simulink model "simulation"  (R2013a)
settings: Solver=ode45  StartTime=0.0  StopTime=10.0  RelTol=1e-3
libraries: elec_lib x72, nesl_utility x5, fl_lib x4, simulink x3, powerlib x1
settings Model: Creator=Fuad  LastModifiedBy=Fuad

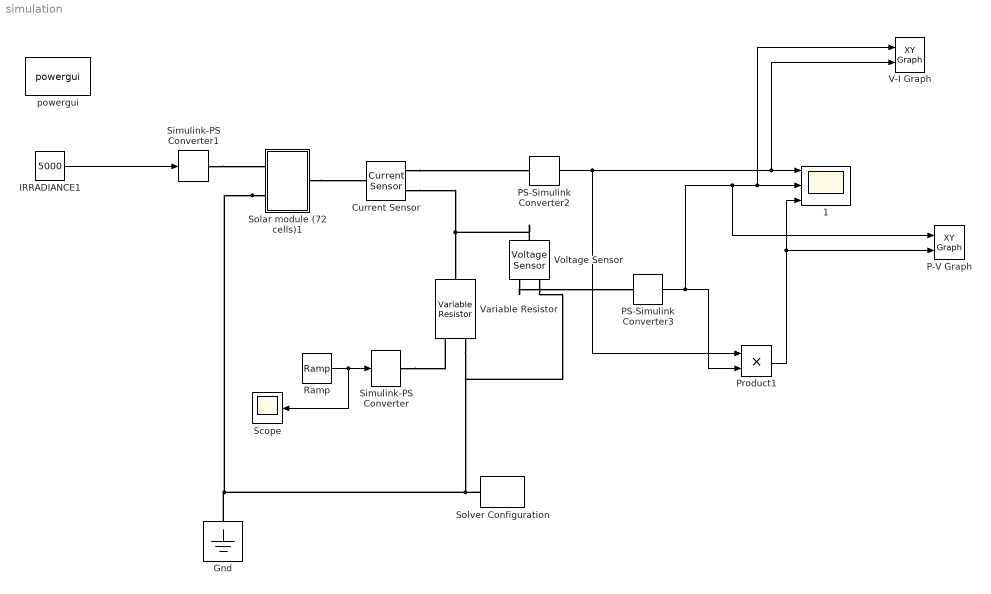
== system simulation ==
  " 1" : Scope  NumInputPorts=3
      settings: TickLabels=on  TimeRange=10  YMin=-5~-5~-5  YMax=5~5~5  SaveName=Sc
  Current Sensor : fl_lib/Electrical/Electrical Sensors/Current Sensor  i1_Log=off  v1_Log=off  LocalVarNames=|i1|v1  LocalVarDescs=|i1|v1  LocalVarLogging=[0 0]
  Gnd : fl_lib/Electrical/Electrical Elements/Electrical Reference  i_Log=off  LocalVarNames=|i  LocalVarDescs=|i  LocalVarLogging=0
  IRRADIANCE1 : Constant  Value=5000
  "P-V Graph " : simulink/Sinks/XY Graph  xmin=0  xmax=50  ymin=0  ymax=900  st=1
  PS-Simulink Converter2 : nesl_utility/PS-Simulink Converter  PhysicalDomain=network_engine_domain  SubClassName=ps_output  LeftPortType=input  RightPortType=output  PseudoPeriodic=off  Frequencies=[]  Unit=1  AffineConversion=off
  PS-Simulink Converter3 : nesl_utility/PS-Simulink Converter  PhysicalDomain=network_engine_domain  SubClassName=ps_output  LeftPortType=input  RightPortType=output  PseudoPeriodic=off  Frequencies=[]  Unit=1  AffineConversion=off
  Product1 : Product
  Ramp : simulink/Sources/Ramp  slope=1  start=0  X0=0
  Scope : Scope
  Simulink-PS Converter : nesl_utility/Simulink-PS Converter  PhysicalDomain=network_engine_domain  SubClassName=ps_input  LeftPortType=input  RightPortType=output  PseudoPeriodic=off  Frequencies=[]  NoiseDistribution=none  NoiseParameters=[]  Unit=1  AffineConversion=off  InputFiltering=on  SimscapeFilterOrder=1  InputFilterTimeConstant=0.001  UdotUserProvided=1
  Simulink-PS Converter1 : nesl_utility/Simulink-PS Converter  PhysicalDomain=network_engine_domain  SubClassName=ps_input  LeftPortType=input  RightPortType=output  PseudoPeriodic=off  Frequencies=[]  NoiseDistribution=none  NoiseParameters=[]  Unit=1  AffineConversion=off  InputFiltering=off  SimscapeFilterOrder=1  InputFilterTimeConstant=.001  UdotUserProvided=0
  Solar module (72 cells)1 : Subsystem
  Solver Configuration : nesl_utility/Solver Configuration  PhysicalDomain=network_engine_domain  SubClassName=solver  LeftPortType=input  RightPortType=generic  Accelerate=off  Tones=[]  Harmonics=[]  SimulateNoise=off  Profile=off  UseLocalSampling=off  EnableSwitchedLinearOptims=on  FrequencyDomain=off  UseCCode=off  UseNewInitialization=off  DoDC=off  ResidualTolerance=1e-09  UseLocalSolver=off  LocalSolverChoice=NE_BACKWARD_EULER_ADVANCER  LocalSolverSampleTime=0.001  DoFixedCost=off  MaxNonlinIter=3  MaxModeIter=2  LinearAlgebra=Sparse  DelaysMemoryBudget=1024
  "V-I Graph " : simulink/Sinks/XY Graph  xmin=0  xmax=50  ymin=0  ymax=100  st=1
  Variable Resistor : fl_lib/Electrical/Electrical Elements/Variable Resistor  Rmin=0 Ohm  i_Log=off  v_Log=off  LocalVarNames=|i|v  LocalVarDescs=|i|v  LocalVarLogging=[0 0]
  Voltage Sensor : fl_lib/Electrical/Electrical Sensors/Voltage Sensor  i1_Log=off  v1_Log=off  LocalVarNames=|i1|v1  LocalVarDescs=|i1|v1  LocalVarLogging=[0 0]
  powergui : powerlib/powergui  Priority=1  SimulationMode=Continuous  SolverType=Tustin  SampleTime=50e-6  frequency=60  SPID=off  DisableSnubberDevices=off  DisableRonSwitches=off  DisableVfSwitches=off  SwTol=0  Interpol=off  DisplayEquations=off  frequencyindice=0  Pbase=100e6  ErrMax=1e-4  Iterations=50  UnitsV=kV  UnitsW=MW  FunctionMessages=off  echomessages=off  HookPort=off  EnableUseOfTLC=off  x0status=blocks  RestoreLinks=warning  ResistiveCurrentMeasurement=off  Frange=[0:2:500]  Ylog=off  Xlog=on  ShowGrid=off  save=off  variable=ZData  ZoomFFT=off  StartTime=0.0  cycles=1  DisplayStyle=1  fundamental=60  FreqAxis=off  MaxFrequency=1000  frequencyindicesteady=1  RmsSteady=1  display=off  Ts=0  methode=off
  wires:
  IRRADIANCE1/1 -> Simulink-PS Converter1/1
  PS-Simulink Converter2/1 -> Product1/1, "V-I Graph "/2, " 1"/1
  Ramp/1 -> Scope/1, Simulink-PS Converter/1
  Product1/1 -> "P-V Graph "/2, " 1"/3
  PS-Simulink Converter3/1 -> "P-V Graph "/1, "V-I Graph "/1, " 1"/2, Product1/2
  connections:
  Solar module (72 cells)1/LConn2 -- Voltage Sensor/RConn2 -- Variable Resistor/LConn2 -- Solver Configuration/RConn1 -- Gnd/LConn1
  Current Sensor/RConn2 -- Voltage Sensor/LConn1 -- Variable Resistor/RConn1
  Simulink-PS Converter1/RConn1 -- Solar module (72 cells)1/LConn1
  Solar module (72 cells)1/RConn1 -- Current Sensor/LConn1
  Simulink-PS Converter/RConn1 -- Variable Resistor/LConn1
  Current Sensor/RConn1 -- PS-Simulink Converter2/LConn1
  Voltage Sensor/RConn1 -- PS-Simulink Converter3/LConn1

== system simulation/Solar module (72 cells)1 ==
  36 solarceel : Subsystem
  36 solarceel1 : Subsystem
  Ir : PMIOPort  Port=1  Side=Left
  + : PMIOPort  Port=2  Side=Right
  - : PMIOPort  Port=3  Side=Left
  connections:
  Ir/RConn1 -- 36 solarceel/LConn1 -- 36 solarceel1/LConn1
  36 solarceel/RConn1 -- 36 solarceel1/LConn2
  +/RConn1 -- 36 solarceel1/RConn1
  -/RConn1 -- 36 solarceel/LConn2

== system simulation/Solar module (72 cells)1/36 solarceel ==
  18 solar cells : Subsystem
  18 solar cells1 : Subsystem
  Ir : PMIOPort  Port=1  Side=Left
  + : PMIOPort  Port=2  Side=Right
  - : PMIOPort  Port=3  Side=Left
  connections:
  Ir/RConn1 -- 18 solar cells1/LConn1 -- 18 solar cells/LConn1
  18 solar cells/RConn1 -- 18 solar cells1/LConn2
  +/RConn1 -- 18 solar cells1/RConn1
  -/RConn1 -- 18 solar cells/LConn2

== system simulation/Solar module (72 cells)1/36 solarceel1 ==
  18 solar cells : Subsystem
  18 solar cells1 : Subsystem
  Ir : PMIOPort  Port=1  Side=Left
  + : PMIOPort  Port=2  Side=Right
  - : PMIOPort  Port=3  Side=Left
  connections:
  18 solar cells/LConn1 -- Ir/RConn1 -- 18 solar cells1/LConn1
  18 solar cells/RConn1 -- 18 solar cells1/LConn2
  +/RConn1 -- 18 solar cells1/RConn1
  -/RConn1 -- 18 solar cells/LConn2

== system simulation/Solar module (72 cells)1/36 solarceel/18 solar cells ==
  6solarcells : Subsystem
  6solarcells1 : Subsystem
  6solarcells2 : Subsystem
  + : PMIOPort  Port=1  Side=Right
  Ir : PMIOPort  Port=2  Side=Left
  - : PMIOPort  Port=3  Side=Left
  connections:
  Ir/RConn1 -- 6solarcells1/LConn1 -- 6solarcells/LConn1 -- 6solarcells2/LConn1
  6solarcells/RConn1 -- 6solarcells1/LConn2
  6solarcells1/RConn1 -- 6solarcells2/LConn2
  +/RConn1 -- 6solarcells2/RConn1
  -/RConn1 -- 6solarcells/LConn2

== system simulation/Solar module (72 cells)1/36 solarceel/18 solar cells1 ==
  6solarcells : Subsystem
  6solarcells1 : Subsystem
  6solarcells2 : Subsystem
  + : PMIOPort  Port=1  Side=Right
  Ir : PMIOPort  Port=2  Side=Left
  - : PMIOPort  Port=3  Side=Left
  connections:
  6solarcells1/LConn1 -- 6solarcells/LConn1 -- Ir/RConn1 -- 6solarcells2/LConn1
  6solarcells/RConn1 -- 6solarcells1/LConn2
  6solarcells1/RConn1 -- 6solarcells2/LConn2
  +/RConn1 -- 6solarcells2/RConn1
  -/RConn1 -- 6solarcells/LConn2

== system simulation/Solar module (72 cells)1/36 solarceel1/18 solar cells ==
  6solarcells : Subsystem
  6solarcells1 : Subsystem
  6solarcells2 : Subsystem
  + : PMIOPort  Port=1  Side=Right
  Ir : PMIOPort  Port=2  Side=Left
  - : PMIOPort  Port=3  Side=Left
  connections:
  6solarcells1/LConn1 -- 6solarcells/LConn1 -- Ir/RConn1 -- 6solarcells2/LConn1
  6solarcells/RConn1 -- 6solarcells1/LConn2
  6solarcells1/RConn1 -- 6solarcells2/LConn2
  +/RConn1 -- 6solarcells2/RConn1
  -/RConn1 -- 6solarcells/LConn2

== system simulation/Solar module (72 cells)1/36 solarceel1/18 solar cells1 ==
  6solarcells : Subsystem
  6solarcells1 : Subsystem
  6solarcells2 : Subsystem
  + : PMIOPort  Port=1  Side=Right
  Ir : PMIOPort  Port=2  Side=Left
  - : PMIOPort  Port=3  Side=Left
  connections:
  6solarcells1/LConn1 -- 6solarcells/LConn1 -- Ir/RConn1 -- 6solarcells2/LConn1
  6solarcells/RConn1 -- 6solarcells1/LConn2
  6solarcells1/RConn1 -- 6solarcells2/LConn2
  +/RConn1 -- 6solarcells2/RConn1
  -/RConn1 -- 6solarcells/LConn2

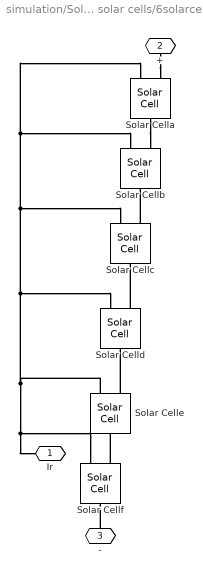
== system simulation/Solar module (72 cells)1/36 solarceel/18 solar cells/6solarcells ==
  Solar Cella : elec_lib/Sources/Solar Cell  prm=1  Isc=4.75 A  Voc=0.6 V  Is=1e-6 A  Is2=0 A  Iph=7.34 A  Ir0=1000 W/m^2  ec=1.6  N2=2  Rs=5.1e-3 Ohm  Rp=Inf Ohm  TIPH1=0.65e-3 1/K  EG=1.12 eV  TXIS1=3  TXIS2=3  TRS1=0  TRP1=0  Tmeas=25 C  TFIXED=25 C  LocalVarLogging=[]  thermal_mass=100 J/K  initial_temperature=25 C
  Solar Cellb : elec_lib/Sources/Solar Cell  prm=1  Isc=4.75 A  Voc=0.6 V  Is=1e-6 A  Is2=0 A  Iph=7.34 A  Ir0=1000 W/m^2  ec=1.6  N2=2  Rs=5.1e-3 Ohm  Rp=Inf Ohm  TIPH1=0.65e-3 1/K  EG=1.12 eV  TXIS1=3  TXIS2=3  TRS1=0  TRP1=0  Tmeas=25 C  TFIXED=25 C  LocalVarLogging=[]  thermal_mass=100 J/K  initial_temperature=25 C
  Solar Cellc : elec_lib/Sources/Solar Cell  prm=1  Isc=4.75 A  Voc=0.6 V  Is=1e-6 A  Is2=0 A  Iph=7.34 A  Ir0=1000 W/m^2  ec=1.6  N2=2  Rs=5.1e-3 Ohm  Rp=Inf Ohm  TIPH1=0.65e-3 1/K  EG=1.12 eV  TXIS1=3  TXIS2=3  TRS1=0  TRP1=0  Tmeas=25 C  TFIXED=25 C  LocalVarLogging=[]  thermal_mass=100 J/K  initial_temperature=25 C
  Solar Celld : elec_lib/Sources/Solar Cell  prm=1  Isc=4.75 A  Voc=0.6 V  Is=1e-6 A  Is2=0 A  Iph=7.34 A  Ir0=1000 W/m^2  ec=1.6  N2=2  Rs=5.1e-3 Ohm  Rp=Inf Ohm  TIPH1=0.65e-3 1/K  EG=1.12 eV  TXIS1=3  TXIS2=3  TRS1=0  TRP1=0  Tmeas=25 C  TFIXED=25 C  LocalVarLogging=[]  thermal_mass=100 J/K  initial_temperature=25 C
  Solar Celle : elec_lib/Sources/Solar Cell  prm=1  Isc=4.75 A  Voc=0.6 V  Is=1e-6 A  Is2=0 A  Iph=7.34 A  Ir0=1000 W/m^2  ec=1.6  N2=2  Rs=5.1e-3 Ohm  Rp=Inf Ohm  TIPH1=0.65e-3 1/K  EG=1.12 eV  TXIS1=3  TXIS2=3  TRS1=0  TRP1=0  Tmeas=25 C  TFIXED=25 C  LocalVarLogging=[]  thermal_mass=100 J/K  initial_temperature=25 C
  Solar Cellf : elec_lib/Sources/Solar Cell  prm=1  Isc=4.75 A  Voc=0.6 V  Is=1e-6 A  Is2=0 A  Iph=7.34 A  Ir0=1000 W/m^2  ec=1.6  N2=2  Rs=5.1e-3 Ohm  Rp=Inf Ohm  TIPH1=0.65e-3 1/K  EG=1.12 eV  TXIS1=3  TXIS2=3  TRS1=0  TRP1=0  Tmeas=25 C  TFIXED=25 C  LocalVarLogging=[]  thermal_mass=100 J/K  initial_temperature=25 C
  Ir : PMIOPort  Port=1  Side=Left
  + : PMIOPort  Port=2  Side=Right
  - : PMIOPort  Port=3  Side=Left
  connections:
  Ir/RConn1 -- Solar Celle/LConn1 -- Solar Celld/LConn1 -- Solar Cellc/LConn1 -- Solar Cellb/LConn1 -- Solar Cella/LConn1 -- Solar Cellf/LConn1
  Solar Cella/RConn1 -- Solar Cellb/LConn2
  Solar Cellc/LConn2 -- Solar Cellb/RConn1
  Solar Celld/LConn2 -- Solar Cellc/RConn1
  Solar Celle/LConn2 -- Solar Celld/RConn1
  Solar Cellf/LConn2 -- Solar Celle/RConn1
  +/RConn1 -- Solar Cella/LConn2
  -/RConn1 -- Solar Cellf/RConn1

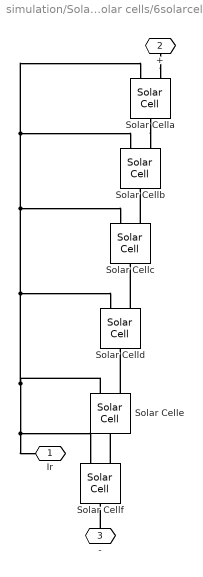
== system simulation/Solar module (72 cells)1/36 solarceel/18 solar cells/6solarcells1 ==
  Solar Cella : elec_lib/Sources/Solar Cell  prm=1  Isc=4.75 A  Voc=0.6 V  Is=1e-6 A  Is2=0 A  Iph=7.34 A  Ir0=1000 W/m^2  ec=1.6  N2=2  Rs=5.1e-3 Ohm  Rp=Inf Ohm  TIPH1=0.65e-3 1/K  EG=1.12 eV  TXIS1=3  TXIS2=3  TRS1=0  TRP1=0  Tmeas=25 C  TFIXED=25 C  LocalVarLogging=[]  thermal_mass=100 J/K  initial_temperature=25 C
  Solar Cellb : elec_lib/Sources/Solar Cell  prm=1  Isc=4.75 A  Voc=0.6 V  Is=1e-6 A  Is2=0 A  Iph=7.34 A  Ir0=1000 W/m^2  ec=1.6  N2=2  Rs=5.1e-3 Ohm  Rp=Inf Ohm  TIPH1=0.65e-3 1/K  EG=1.12 eV  TXIS1=3  TXIS2=3  TRS1=0  TRP1=0  Tmeas=25 C  TFIXED=25 C  LocalVarLogging=[]  thermal_mass=100 J/K  initial_temperature=25 C
  Solar Cellc : elec_lib/Sources/Solar Cell  prm=1  Isc=4.75 A  Voc=0.6 V  Is=1e-6 A  Is2=0 A  Iph=7.34 A  Ir0=1000 W/m^2  ec=1.6  N2=2  Rs=5.1e-3 Ohm  Rp=Inf Ohm  TIPH1=0.65e-3 1/K  EG=1.12 eV  TXIS1=3  TXIS2=3  TRS1=0  TRP1=0  Tmeas=25 C  TFIXED=25 C  LocalVarLogging=[]  thermal_mass=100 J/K  initial_temperature=25 C
  Solar Celld : elec_lib/Sources/Solar Cell  prm=1  Isc=4.75 A  Voc=0.6 V  Is=1e-6 A  Is2=0 A  Iph=7.34 A  Ir0=1000 W/m^2  ec=1.6  N2=2  Rs=5.1e-3 Ohm  Rp=Inf Ohm  TIPH1=0.65e-3 1/K  EG=1.12 eV  TXIS1=3  TXIS2=3  TRS1=0  TRP1=0  Tmeas=25 C  TFIXED=25 C  LocalVarLogging=[]  thermal_mass=100 J/K  initial_temperature=25 C
  Solar Celle : elec_lib/Sources/Solar Cell  prm=1  Isc=4.75 A  Voc=0.6 V  Is=1e-6 A  Is2=0 A  Iph=7.34 A  Ir0=1000 W/m^2  ec=1.6  N2=2  Rs=5.1e-3 Ohm  Rp=Inf Ohm  TIPH1=0.65e-3 1/K  EG=1.12 eV  TXIS1=3  TXIS2=3  TRS1=0  TRP1=0  Tmeas=25 C  TFIXED=25 C  LocalVarLogging=[]  thermal_mass=100 J/K  initial_temperature=25 C
  Solar Cellf : elec_lib/Sources/Solar Cell  prm=1  Isc=4.75 A  Voc=0.6 V  Is=1e-6 A  Is2=0 A  Iph=7.34 A  Ir0=1000 W/m^2  ec=1.6  N2=2  Rs=5.1e-3 Ohm  Rp=Inf Ohm  TIPH1=0.65e-3 1/K  EG=1.12 eV  TXIS1=3  TXIS2=3  TRS1=0  TRP1=0  Tmeas=25 C  TFIXED=25 C  LocalVarLogging=[]  thermal_mass=100 J/K  initial_temperature=25 C
  Ir : PMIOPort  Port=1  Side=Left
  + : PMIOPort  Port=2  Side=Right
  - : PMIOPort  Port=3  Side=Left
  connections:
  Solar Celle/LConn1 -- Solar Cellf/LConn1 -- Ir/RConn1 -- Solar Celld/LConn1 -- Solar Cellc/LConn1 -- Solar Cella/LConn1 -- Solar Cellb/LConn1
  Solar Cella/RConn1 -- Solar Cellb/LConn2
  Solar Cellc/LConn2 -- Solar Cellb/RConn1
  Solar Celld/LConn2 -- Solar Cellc/RConn1
  Solar Celle/LConn2 -- Solar Celld/RConn1
  Solar Cellf/LConn2 -- Solar Celle/RConn1
  +/RConn1 -- Solar Cella/LConn2
  -/RConn1 -- Solar Cellf/RConn1

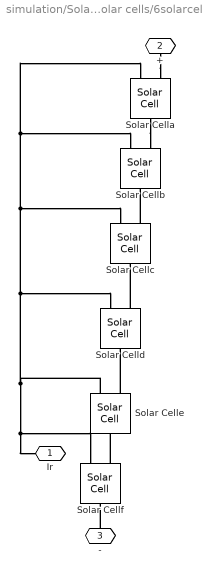
== system simulation/Solar module (72 cells)1/36 solarceel/18 solar cells/6solarcells2 ==
  Solar Cella : elec_lib/Sources/Solar Cell  prm=1  Isc=4.75 A  Voc=0.6 V  Is=1e-6 A  Is2=0 A  Iph=7.34 A  Ir0=1000 W/m^2  ec=1.6  N2=2  Rs=5.1e-3 Ohm  Rp=Inf Ohm  TIPH1=0.65e-3 1/K  EG=1.12 eV  TXIS1=3  TXIS2=3  TRS1=0  TRP1=0  Tmeas=25 C  TFIXED=25 C  LocalVarLogging=[]  thermal_mass=100 J/K  initial_temperature=25 C
  Solar Cellb : elec_lib/Sources/Solar Cell  prm=1  Isc=4.75 A  Voc=0.6 V  Is=1e-6 A  Is2=0 A  Iph=7.34 A  Ir0=1000 W/m^2  ec=1.6  N2=2  Rs=5.1e-3 Ohm  Rp=Inf Ohm  TIPH1=0.65e-3 1/K  EG=1.12 eV  TXIS1=3  TXIS2=3  TRS1=0  TRP1=0  Tmeas=25 C  TFIXED=25 C  LocalVarLogging=[]  thermal_mass=100 J/K  initial_temperature=25 C
  Solar Cellc : elec_lib/Sources/Solar Cell  prm=1  Isc=4.75 A  Voc=0.6 V  Is=1e-6 A  Is2=0 A  Iph=7.34 A  Ir0=1000 W/m^2  ec=1.6  N2=2  Rs=5.1e-3 Ohm  Rp=Inf Ohm  TIPH1=0.65e-3 1/K  EG=1.12 eV  TXIS1=3  TXIS2=3  TRS1=0  TRP1=0  Tmeas=25 C  TFIXED=25 C  LocalVarLogging=[]  thermal_mass=100 J/K  initial_temperature=25 C
  Solar Celld : elec_lib/Sources/Solar Cell  prm=1  Isc=4.75 A  Voc=0.6 V  Is=1e-6 A  Is2=0 A  Iph=7.34 A  Ir0=1000 W/m^2  ec=1.6  N2=2  Rs=5.1e-3 Ohm  Rp=Inf Ohm  TIPH1=0.65e-3 1/K  EG=1.12 eV  TXIS1=3  TXIS2=3  TRS1=0  TRP1=0  Tmeas=25 C  TFIXED=25 C  LocalVarLogging=[]  thermal_mass=100 J/K  initial_temperature=25 C
  Solar Celle : elec_lib/Sources/Solar Cell  prm=1  Isc=4.75 A  Voc=0.6 V  Is=1e-6 A  Is2=0 A  Iph=7.34 A  Ir0=1000 W/m^2  ec=1.6  N2=2  Rs=5.1e-3 Ohm  Rp=Inf Ohm  TIPH1=0.65e-3 1/K  EG=1.12 eV  TXIS1=3  TXIS2=3  TRS1=0  TRP1=0  Tmeas=25 C  TFIXED=25 C  LocalVarLogging=[]  thermal_mass=100 J/K  initial_temperature=25 C
  Solar Cellf : elec_lib/Sources/Solar Cell  prm=1  Isc=4.75 A  Voc=0.6 V  Is=1e-6 A  Is2=0 A  Iph=7.34 A  Ir0=1000 W/m^2  ec=1.6  N2=2  Rs=5.1e-3 Ohm  Rp=Inf Ohm  TIPH1=0.65e-3 1/K  EG=1.12 eV  TXIS1=3  TXIS2=3  TRS1=0  TRP1=0  Tmeas=25 C  TFIXED=25 C  LocalVarLogging=[]  thermal_mass=100 J/K  initial_temperature=25 C
  Ir : PMIOPort  Port=1  Side=Left
  + : PMIOPort  Port=2  Side=Right
  - : PMIOPort  Port=3  Side=Left
  connections:
  Solar Celle/LConn1 -- Solar Cellf/LConn1 -- Ir/RConn1 -- Solar Celld/LConn1 -- Solar Cellc/LConn1 -- Solar Cella/LConn1 -- Solar Cellb/LConn1
  Solar Cella/RConn1 -- Solar Cellb/LConn2
  Solar Cellc/LConn2 -- Solar Cellb/RConn1
  Solar Celld/LConn2 -- Solar Cellc/RConn1
  Solar Celle/LConn2 -- Solar Celld/RConn1
  Solar Cellf/LConn2 -- Solar Celle/RConn1
  +/RConn1 -- Solar Cella/LConn2
  -/RConn1 -- Solar Cellf/RConn1

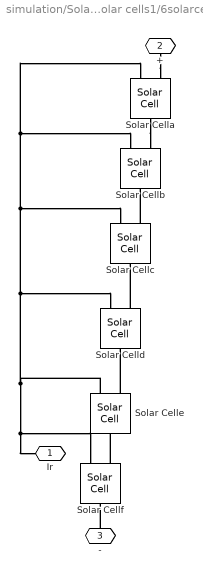
== system simulation/Solar module (72 cells)1/36 solarceel/18 solar cells1/6solarcells ==
  Solar Cella : elec_lib/Sources/Solar Cell  prm=1  Isc=4.75 A  Voc=0.6 V  Is=1e-6 A  Is2=0 A  Iph=7.34 A  Ir0=1000 W/m^2  ec=1.6  N2=2  Rs=5.1e-3 Ohm  Rp=Inf Ohm  TIPH1=0.65e-3 1/K  EG=1.12 eV  TXIS1=3  TXIS2=3  TRS1=0  TRP1=0  Tmeas=25 C  TFIXED=25 C  LocalVarLogging=[]  thermal_mass=100 J/K  initial_temperature=25 C
  Solar Cellb : elec_lib/Sources/Solar Cell  prm=1  Isc=4.75 A  Voc=0.6 V  Is=1e-6 A  Is2=0 A  Iph=7.34 A  Ir0=1000 W/m^2  ec=1.6  N2=2  Rs=5.1e-3 Ohm  Rp=Inf Ohm  TIPH1=0.65e-3 1/K  EG=1.12 eV  TXIS1=3  TXIS2=3  TRS1=0  TRP1=0  Tmeas=25 C  TFIXED=25 C  LocalVarLogging=[]  thermal_mass=100 J/K  initial_temperature=25 C
  Solar Cellc : elec_lib/Sources/Solar Cell  prm=1  Isc=4.75 A  Voc=0.6 V  Is=1e-6 A  Is2=0 A  Iph=7.34 A  Ir0=1000 W/m^2  ec=1.6  N2=2  Rs=5.1e-3 Ohm  Rp=Inf Ohm  TIPH1=0.65e-3 1/K  EG=1.12 eV  TXIS1=3  TXIS2=3  TRS1=0  TRP1=0  Tmeas=25 C  TFIXED=25 C  LocalVarLogging=[]  thermal_mass=100 J/K  initial_temperature=25 C
  Solar Celld : elec_lib/Sources/Solar Cell  prm=1  Isc=4.75 A  Voc=0.6 V  Is=1e-6 A  Is2=0 A  Iph=7.34 A  Ir0=1000 W/m^2  ec=1.6  N2=2  Rs=5.1e-3 Ohm  Rp=Inf Ohm  TIPH1=0.65e-3 1/K  EG=1.12 eV  TXIS1=3  TXIS2=3  TRS1=0  TRP1=0  Tmeas=25 C  TFIXED=25 C  LocalVarLogging=[]  thermal_mass=100 J/K  initial_temperature=25 C
  Solar Celle : elec_lib/Sources/Solar Cell  prm=1  Isc=4.75 A  Voc=0.6 V  Is=1e-6 A  Is2=0 A  Iph=7.34 A  Ir0=1000 W/m^2  ec=1.6  N2=2  Rs=5.1e-3 Ohm  Rp=Inf Ohm  TIPH1=0.65e-3 1/K  EG=1.12 eV  TXIS1=3  TXIS2=3  TRS1=0  TRP1=0  Tmeas=25 C  TFIXED=25 C  LocalVarLogging=[]  thermal_mass=100 J/K  initial_temperature=25 C
  Solar Cellf : elec_lib/Sources/Solar Cell  prm=1  Isc=4.75 A  Voc=0.6 V  Is=1e-6 A  Is2=0 A  Iph=7.34 A  Ir0=1000 W/m^2  ec=1.6  N2=2  Rs=5.1e-3 Ohm  Rp=Inf Ohm  TIPH1=0.65e-3 1/K  EG=1.12 eV  TXIS1=3  TXIS2=3  TRS1=0  TRP1=0  Tmeas=25 C  TFIXED=25 C  LocalVarLogging=[]  thermal_mass=100 J/K  initial_temperature=25 C
  Ir : PMIOPort  Port=1  Side=Left
  + : PMIOPort  Port=2  Side=Right
  - : PMIOPort  Port=3  Side=Left
  connections:
  Solar Celle/LConn1 -- Solar Cellf/LConn1 -- Ir/RConn1 -- Solar Celld/LConn1 -- Solar Cellc/LConn1 -- Solar Cella/LConn1 -- Solar Cellb/LConn1
  Solar Cella/RConn1 -- Solar Cellb/LConn2
  Solar Cellc/LConn2 -- Solar Cellb/RConn1
  Solar Celld/LConn2 -- Solar Cellc/RConn1
  Solar Celle/LConn2 -- Solar Celld/RConn1
  Solar Cellf/LConn2 -- Solar Celle/RConn1
  +/RConn1 -- Solar Cella/LConn2
  -/RConn1 -- Solar Cellf/RConn1

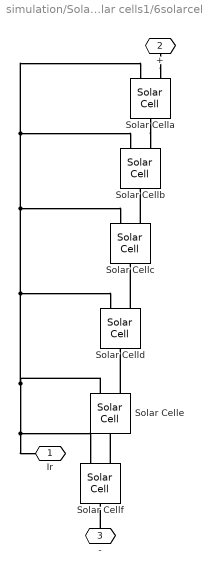
== system simulation/Solar module (72 cells)1/36 solarceel/18 solar cells1/6solarcells1 ==
  Solar Cella : elec_lib/Sources/Solar Cell  prm=1  Isc=4.75 A  Voc=0.6 V  Is=1e-6 A  Is2=0 A  Iph=7.34 A  Ir0=1000 W/m^2  ec=1.6  N2=2  Rs=5.1e-3 Ohm  Rp=Inf Ohm  TIPH1=0.65e-3 1/K  EG=1.12 eV  TXIS1=3  TXIS2=3  TRS1=0  TRP1=0  Tmeas=25 C  TFIXED=25 C  LocalVarLogging=[]  thermal_mass=100 J/K  initial_temperature=25 C
  Solar Cellb : elec_lib/Sources/Solar Cell  prm=1  Isc=4.75 A  Voc=0.6 V  Is=1e-6 A  Is2=0 A  Iph=7.34 A  Ir0=1000 W/m^2  ec=1.6  N2=2  Rs=5.1e-3 Ohm  Rp=Inf Ohm  TIPH1=0.65e-3 1/K  EG=1.12 eV  TXIS1=3  TXIS2=3  TRS1=0  TRP1=0  Tmeas=25 C  TFIXED=25 C  LocalVarLogging=[]  thermal_mass=100 J/K  initial_temperature=25 C
  Solar Cellc : elec_lib/Sources/Solar Cell  prm=1  Isc=4.75 A  Voc=0.6 V  Is=1e-6 A  Is2=0 A  Iph=7.34 A  Ir0=1000 W/m^2  ec=1.6  N2=2  Rs=5.1e-3 Ohm  Rp=Inf Ohm  TIPH1=0.65e-3 1/K  EG=1.12 eV  TXIS1=3  TXIS2=3  TRS1=0  TRP1=0  Tmeas=25 C  TFIXED=25 C  LocalVarLogging=[]  thermal_mass=100 J/K  initial_temperature=25 C
  Solar Celld : elec_lib/Sources/Solar Cell  prm=1  Isc=4.75 A  Voc=0.6 V  Is=1e-6 A  Is2=0 A  Iph=7.34 A  Ir0=1000 W/m^2  ec=1.6  N2=2  Rs=5.1e-3 Ohm  Rp=Inf Ohm  TIPH1=0.65e-3 1/K  EG=1.12 eV  TXIS1=3  TXIS2=3  TRS1=0  TRP1=0  Tmeas=25 C  TFIXED=25 C  LocalVarLogging=[]  thermal_mass=100 J/K  initial_temperature=25 C
  Solar Celle : elec_lib/Sources/Solar Cell  prm=1  Isc=4.75 A  Voc=0.6 V  Is=1e-6 A  Is2=0 A  Iph=7.34 A  Ir0=1000 W/m^2  ec=1.6  N2=2  Rs=5.1e-3 Ohm  Rp=Inf Ohm  TIPH1=0.65e-3 1/K  EG=1.12 eV  TXIS1=3  TXIS2=3  TRS1=0  TRP1=0  Tmeas=25 C  TFIXED=25 C  LocalVarLogging=[]  thermal_mass=100 J/K  initial_temperature=25 C
  Solar Cellf : elec_lib/Sources/Solar Cell  prm=1  Isc=4.75 A  Voc=0.6 V  Is=1e-6 A  Is2=0 A  Iph=7.34 A  Ir0=1000 W/m^2  ec=1.6  N2=2  Rs=5.1e-3 Ohm  Rp=Inf Ohm  TIPH1=0.65e-3 1/K  EG=1.12 eV  TXIS1=3  TXIS2=3  TRS1=0  TRP1=0  Tmeas=25 C  TFIXED=25 C  LocalVarLogging=[]  thermal_mass=100 J/K  initial_temperature=25 C
  Ir : PMIOPort  Port=1  Side=Left
  + : PMIOPort  Port=2  Side=Right
  - : PMIOPort  Port=3  Side=Left
  connections:
  Solar Celle/LConn1 -- Solar Cellf/LConn1 -- Ir/RConn1 -- Solar Celld/LConn1 -- Solar Cellc/LConn1 -- Solar Cella/LConn1 -- Solar Cellb/LConn1
  Solar Cella/RConn1 -- Solar Cellb/LConn2
  Solar Cellc/LConn2 -- Solar Cellb/RConn1
  Solar Celld/LConn2 -- Solar Cellc/RConn1
  Solar Celle/LConn2 -- Solar Celld/RConn1
  Solar Cellf/LConn2 -- Solar Celle/RConn1
  +/RConn1 -- Solar Cella/LConn2
  -/RConn1 -- Solar Cellf/RConn1

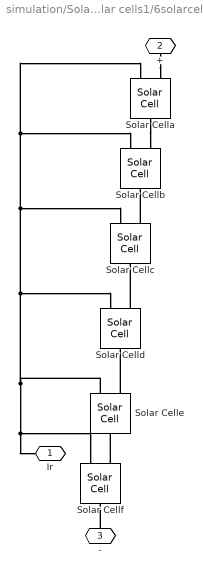
== system simulation/Solar module (72 cells)1/36 solarceel/18 solar cells1/6solarcells2 ==
  Solar Cella : elec_lib/Sources/Solar Cell  prm=1  Isc=4.75 A  Voc=0.6 V  Is=1e-6 A  Is2=0 A  Iph=7.34 A  Ir0=1000 W/m^2  ec=1.6  N2=2  Rs=5.1e-3 Ohm  Rp=Inf Ohm  TIPH1=0.65e-3 1/K  EG=1.12 eV  TXIS1=3  TXIS2=3  TRS1=0  TRP1=0  Tmeas=25 C  TFIXED=25 C  LocalVarLogging=[]  thermal_mass=100 J/K  initial_temperature=25 C
  Solar Cellb : elec_lib/Sources/Solar Cell  prm=1  Isc=4.75 A  Voc=0.6 V  Is=1e-6 A  Is2=0 A  Iph=7.34 A  Ir0=1000 W/m^2  ec=1.6  N2=2  Rs=5.1e-3 Ohm  Rp=Inf Ohm  TIPH1=0.65e-3 1/K  EG=1.12 eV  TXIS1=3  TXIS2=3  TRS1=0  TRP1=0  Tmeas=25 C  TFIXED=25 C  LocalVarLogging=[]  thermal_mass=100 J/K  initial_temperature=25 C
  Solar Cellc : elec_lib/Sources/Solar Cell  prm=1  Isc=4.75 A  Voc=0.6 V  Is=1e-6 A  Is2=0 A  Iph=7.34 A  Ir0=1000 W/m^2  ec=1.6  N2=2  Rs=5.1e-3 Ohm  Rp=Inf Ohm  TIPH1=0.65e-3 1/K  EG=1.12 eV  TXIS1=3  TXIS2=3  TRS1=0  TRP1=0  Tmeas=25 C  TFIXED=25 C  LocalVarLogging=[]  thermal_mass=100 J/K  initial_temperature=25 C
  Solar Celld : elec_lib/Sources/Solar Cell  prm=1  Isc=4.75 A  Voc=0.6 V  Is=1e-6 A  Is2=0 A  Iph=7.34 A  Ir0=1000 W/m^2  ec=1.6  N2=2  Rs=5.1e-3 Ohm  Rp=Inf Ohm  TIPH1=0.65e-3 1/K  EG=1.12 eV  TXIS1=3  TXIS2=3  TRS1=0  TRP1=0  Tmeas=25 C  TFIXED=25 C  LocalVarLogging=[]  thermal_mass=100 J/K  initial_temperature=25 C
  Solar Celle : elec_lib/Sources/Solar Cell  prm=1  Isc=4.75 A  Voc=0.6 V  Is=1e-6 A  Is2=0 A  Iph=7.34 A  Ir0=1000 W/m^2  ec=1.6  N2=2  Rs=5.1e-3 Ohm  Rp=Inf Ohm  TIPH1=0.65e-3 1/K  EG=1.12 eV  TXIS1=3  TXIS2=3  TRS1=0  TRP1=0  Tmeas=25 C  TFIXED=25 C  LocalVarLogging=[]  thermal_mass=100 J/K  initial_temperature=25 C
  Solar Cellf : elec_lib/Sources/Solar Cell  prm=1  Isc=4.75 A  Voc=0.6 V  Is=1e-6 A  Is2=0 A  Iph=7.34 A  Ir0=1000 W/m^2  ec=1.6  N2=2  Rs=5.1e-3 Ohm  Rp=Inf Ohm  TIPH1=0.65e-3 1/K  EG=1.12 eV  TXIS1=3  TXIS2=3  TRS1=0  TRP1=0  Tmeas=25 C  TFIXED=25 C  LocalVarLogging=[]  thermal_mass=100 J/K  initial_temperature=25 C
  Ir : PMIOPort  Port=1  Side=Left
  + : PMIOPort  Port=2  Side=Right
  - : PMIOPort  Port=3  Side=Left
  connections:
  Solar Celle/LConn1 -- Solar Cellf/LConn1 -- Ir/RConn1 -- Solar Celld/LConn1 -- Solar Cellc/LConn1 -- Solar Cella/LConn1 -- Solar Cellb/LConn1
  Solar Cella/RConn1 -- Solar Cellb/LConn2
  Solar Cellc/LConn2 -- Solar Cellb/RConn1
  Solar Celld/LConn2 -- Solar Cellc/RConn1
  Solar Celle/LConn2 -- Solar Celld/RConn1
  Solar Cellf/LConn2 -- Solar Celle/RConn1
  +/RConn1 -- Solar Cella/LConn2
  -/RConn1 -- Solar Cellf/RConn1

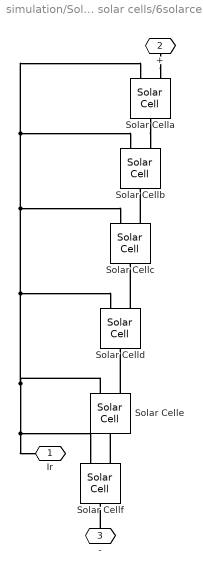
== system simulation/Solar module (72 cells)1/36 solarceel1/18 solar cells/6solarcells ==
  Solar Cella : elec_lib/Sources/Solar Cell  prm=1  Isc=4.75 A  Voc=0.6 V  Is=1e-6 A  Is2=0 A  Iph=7.34 A  Ir0=1000 W/m^2  ec=1.6  N2=2  Rs=5.1e-3 Ohm  Rp=Inf Ohm  TIPH1=0.65e-3 1/K  EG=1.12 eV  TXIS1=3  TXIS2=3  TRS1=0  TRP1=0  Tmeas=25 C  TFIXED=25 C  LocalVarLogging=[]  thermal_mass=100 J/K  initial_temperature=25 C
  Solar Cellb : elec_lib/Sources/Solar Cell  prm=1  Isc=4.75 A  Voc=0.6 V  Is=1e-6 A  Is2=0 A  Iph=7.34 A  Ir0=1000 W/m^2  ec=1.6  N2=2  Rs=5.1e-3 Ohm  Rp=Inf Ohm  TIPH1=0.65e-3 1/K  EG=1.12 eV  TXIS1=3  TXIS2=3  TRS1=0  TRP1=0  Tmeas=25 C  TFIXED=25 C  LocalVarLogging=[]  thermal_mass=100 J/K  initial_temperature=25 C
  Solar Cellc : elec_lib/Sources/Solar Cell  prm=1  Isc=4.75 A  Voc=0.6 V  Is=1e-6 A  Is2=0 A  Iph=7.34 A  Ir0=1000 W/m^2  ec=1.6  N2=2  Rs=5.1e-3 Ohm  Rp=Inf Ohm  TIPH1=0.65e-3 1/K  EG=1.12 eV  TXIS1=3  TXIS2=3  TRS1=0  TRP1=0  Tmeas=25 C  TFIXED=25 C  LocalVarLogging=[]  thermal_mass=100 J/K  initial_temperature=25 C
  Solar Celld : elec_lib/Sources/Solar Cell  prm=1  Isc=4.75 A  Voc=0.6 V  Is=1e-6 A  Is2=0 A  Iph=7.34 A  Ir0=1000 W/m^2  ec=1.6  N2=2  Rs=5.1e-3 Ohm  Rp=Inf Ohm  TIPH1=0.65e-3 1/K  EG=1.12 eV  TXIS1=3  TXIS2=3  TRS1=0  TRP1=0  Tmeas=25 C  TFIXED=25 C  LocalVarLogging=[]  thermal_mass=100 J/K  initial_temperature=25 C
  Solar Celle : elec_lib/Sources/Solar Cell  prm=1  Isc=4.75 A  Voc=0.6 V  Is=1e-6 A  Is2=0 A  Iph=7.34 A  Ir0=1000 W/m^2  ec=1.6  N2=2  Rs=5.1e-3 Ohm  Rp=Inf Ohm  TIPH1=0.65e-3 1/K  EG=1.12 eV  TXIS1=3  TXIS2=3  TRS1=0  TRP1=0  Tmeas=25 C  TFIXED=25 C  LocalVarLogging=[]  thermal_mass=100 J/K  initial_temperature=25 C
  Solar Cellf : elec_lib/Sources/Solar Cell  prm=1  Isc=4.75 A  Voc=0.6 V  Is=1e-6 A  Is2=0 A  Iph=7.34 A  Ir0=1000 W/m^2  ec=1.6  N2=2  Rs=5.1e-3 Ohm  Rp=Inf Ohm  TIPH1=0.65e-3 1/K  EG=1.12 eV  TXIS1=3  TXIS2=3  TRS1=0  TRP1=0  Tmeas=25 C  TFIXED=25 C  LocalVarLogging=[]  thermal_mass=100 J/K  initial_temperature=25 C
  Ir : PMIOPort  Port=1  Side=Left
  + : PMIOPort  Port=2  Side=Right
  - : PMIOPort  Port=3  Side=Left
  connections:
  Solar Celle/LConn1 -- Solar Cellf/LConn1 -- Ir/RConn1 -- Solar Celld/LConn1 -- Solar Cellc/LConn1 -- Solar Cella/LConn1 -- Solar Cellb/LConn1
  Solar Cella/RConn1 -- Solar Cellb/LConn2
  Solar Cellc/LConn2 -- Solar Cellb/RConn1
  Solar Celld/LConn2 -- Solar Cellc/RConn1
  Solar Celle/LConn2 -- Solar Celld/RConn1
  Solar Cellf/LConn2 -- Solar Celle/RConn1
  +/RConn1 -- Solar Cella/LConn2
  -/RConn1 -- Solar Cellf/RConn1

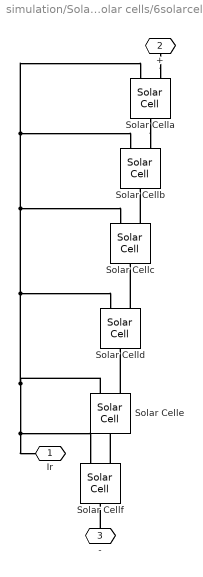
== system simulation/Solar module (72 cells)1/36 solarceel1/18 solar cells/6solarcells1 ==
  Solar Cella : elec_lib/Sources/Solar Cell  prm=1  Isc=4.75 A  Voc=0.6 V  Is=1e-6 A  Is2=0 A  Iph=7.34 A  Ir0=1000 W/m^2  ec=1.6  N2=2  Rs=5.1e-3 Ohm  Rp=Inf Ohm  TIPH1=0.65e-3 1/K  EG=1.12 eV  TXIS1=3  TXIS2=3  TRS1=0  TRP1=0  Tmeas=25 C  TFIXED=25 C  LocalVarLogging=[]  thermal_mass=100 J/K  initial_temperature=25 C
  Solar Cellb : elec_lib/Sources/Solar Cell  prm=1  Isc=4.75 A  Voc=0.6 V  Is=1e-6 A  Is2=0 A  Iph=7.34 A  Ir0=1000 W/m^2  ec=1.6  N2=2  Rs=5.1e-3 Ohm  Rp=Inf Ohm  TIPH1=0.65e-3 1/K  EG=1.12 eV  TXIS1=3  TXIS2=3  TRS1=0  TRP1=0  Tmeas=25 C  TFIXED=25 C  LocalVarLogging=[]  thermal_mass=100 J/K  initial_temperature=25 C
  Solar Cellc : elec_lib/Sources/Solar Cell  prm=1  Isc=4.75 A  Voc=0.6 V  Is=1e-6 A  Is2=0 A  Iph=7.34 A  Ir0=1000 W/m^2  ec=1.6  N2=2  Rs=5.1e-3 Ohm  Rp=Inf Ohm  TIPH1=0.65e-3 1/K  EG=1.12 eV  TXIS1=3  TXIS2=3  TRS1=0  TRP1=0  Tmeas=25 C  TFIXED=25 C  LocalVarLogging=[]  thermal_mass=100 J/K  initial_temperature=25 C
  Solar Celld : elec_lib/Sources/Solar Cell  prm=1  Isc=4.75 A  Voc=0.6 V  Is=1e-6 A  Is2=0 A  Iph=7.34 A  Ir0=1000 W/m^2  ec=1.6  N2=2  Rs=5.1e-3 Ohm  Rp=Inf Ohm  TIPH1=0.65e-3 1/K  EG=1.12 eV  TXIS1=3  TXIS2=3  TRS1=0  TRP1=0  Tmeas=25 C  TFIXED=25 C  LocalVarLogging=[]  thermal_mass=100 J/K  initial_temperature=25 C
  Solar Celle : elec_lib/Sources/Solar Cell  prm=1  Isc=4.75 A  Voc=0.6 V  Is=1e-6 A  Is2=0 A  Iph=7.34 A  Ir0=1000 W/m^2  ec=1.6  N2=2  Rs=5.1e-3 Ohm  Rp=Inf Ohm  TIPH1=0.65e-3 1/K  EG=1.12 eV  TXIS1=3  TXIS2=3  TRS1=0  TRP1=0  Tmeas=25 C  TFIXED=25 C  LocalVarLogging=[]  thermal_mass=100 J/K  initial_temperature=25 C
  Solar Cellf : elec_lib/Sources/Solar Cell  prm=1  Isc=4.75 A  Voc=0.6 V  Is=1e-6 A  Is2=0 A  Iph=7.34 A  Ir0=1000 W/m^2  ec=1.6  N2=2  Rs=5.1e-3 Ohm  Rp=Inf Ohm  TIPH1=0.65e-3 1/K  EG=1.12 eV  TXIS1=3  TXIS2=3  TRS1=0  TRP1=0  Tmeas=25 C  TFIXED=25 C  LocalVarLogging=[]  thermal_mass=100 J/K  initial_temperature=25 C
  Ir : PMIOPort  Port=1  Side=Left
  + : PMIOPort  Port=2  Side=Right
  - : PMIOPort  Port=3  Side=Left
  connections:
  Solar Celle/LConn1 -- Solar Cellf/LConn1 -- Ir/RConn1 -- Solar Celld/LConn1 -- Solar Cellc/LConn1 -- Solar Cella/LConn1 -- Solar Cellb/LConn1
  Solar Cella/RConn1 -- Solar Cellb/LConn2
  Solar Cellc/LConn2 -- Solar Cellb/RConn1
  Solar Celld/LConn2 -- Solar Cellc/RConn1
  Solar Celle/LConn2 -- Solar Celld/RConn1
  Solar Cellf/LConn2 -- Solar Celle/RConn1
  +/RConn1 -- Solar Cella/LConn2
  -/RConn1 -- Solar Cellf/RConn1

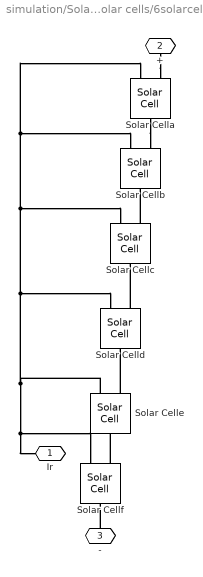
== system simulation/Solar module (72 cells)1/36 solarceel1/18 solar cells/6solarcells2 ==
  Solar Cella : elec_lib/Sources/Solar Cell  prm=1  Isc=4.75 A  Voc=0.6 V  Is=1e-6 A  Is2=0 A  Iph=7.34 A  Ir0=1000 W/m^2  ec=1.6  N2=2  Rs=5.1e-3 Ohm  Rp=Inf Ohm  TIPH1=0.65e-3 1/K  EG=1.12 eV  TXIS1=3  TXIS2=3  TRS1=0  TRP1=0  Tmeas=25 C  TFIXED=25 C  LocalVarLogging=[]  thermal_mass=100 J/K  initial_temperature=25 C
  Solar Cellb : elec_lib/Sources/Solar Cell  prm=1  Isc=4.75 A  Voc=0.6 V  Is=1e-6 A  Is2=0 A  Iph=7.34 A  Ir0=1000 W/m^2  ec=1.6  N2=2  Rs=5.1e-3 Ohm  Rp=Inf Ohm  TIPH1=0.65e-3 1/K  EG=1.12 eV  TXIS1=3  TXIS2=3  TRS1=0  TRP1=0  Tmeas=25 C  TFIXED=25 C  LocalVarLogging=[]  thermal_mass=100 J/K  initial_temperature=25 C
  Solar Cellc : elec_lib/Sources/Solar Cell  prm=1  Isc=4.75 A  Voc=0.6 V  Is=1e-6 A  Is2=0 A  Iph=7.34 A  Ir0=1000 W/m^2  ec=1.6  N2=2  Rs=5.1e-3 Ohm  Rp=Inf Ohm  TIPH1=0.65e-3 1/K  EG=1.12 eV  TXIS1=3  TXIS2=3  TRS1=0  TRP1=0  Tmeas=25 C  TFIXED=25 C  LocalVarLogging=[]  thermal_mass=100 J/K  initial_temperature=25 C
  Solar Celld : elec_lib/Sources/Solar Cell  prm=1  Isc=4.75 A  Voc=0.6 V  Is=1e-6 A  Is2=0 A  Iph=7.34 A  Ir0=1000 W/m^2  ec=1.6  N2=2  Rs=5.1e-3 Ohm  Rp=Inf Ohm  TIPH1=0.65e-3 1/K  EG=1.12 eV  TXIS1=3  TXIS2=3  TRS1=0  TRP1=0  Tmeas=25 C  TFIXED=25 C  LocalVarLogging=[]  thermal_mass=100 J/K  initial_temperature=25 C
  Solar Celle : elec_lib/Sources/Solar Cell  prm=1  Isc=4.75 A  Voc=0.6 V  Is=1e-6 A  Is2=0 A  Iph=7.34 A  Ir0=1000 W/m^2  ec=1.6  N2=2  Rs=5.1e-3 Ohm  Rp=Inf Ohm  TIPH1=0.65e-3 1/K  EG=1.12 eV  TXIS1=3  TXIS2=3  TRS1=0  TRP1=0  Tmeas=25 C  TFIXED=25 C  LocalVarLogging=[]  thermal_mass=100 J/K  initial_temperature=25 C
  Solar Cellf : elec_lib/Sources/Solar Cell  prm=1  Isc=4.75 A  Voc=0.6 V  Is=1e-6 A  Is2=0 A  Iph=7.34 A  Ir0=1000 W/m^2  ec=1.6  N2=2  Rs=5.1e-3 Ohm  Rp=Inf Ohm  TIPH1=0.65e-3 1/K  EG=1.12 eV  TXIS1=3  TXIS2=3  TRS1=0  TRP1=0  Tmeas=25 C  TFIXED=25 C  LocalVarLogging=[]  thermal_mass=100 J/K  initial_temperature=25 C
  Ir : PMIOPort  Port=1  Side=Left
  + : PMIOPort  Port=2  Side=Right
  - : PMIOPort  Port=3  Side=Left
  connections:
  Solar Celle/LConn1 -- Solar Cellf/LConn1 -- Ir/RConn1 -- Solar Celld/LConn1 -- Solar Cellc/LConn1 -- Solar Cella/LConn1 -- Solar Cellb/LConn1
  Solar Cella/RConn1 -- Solar Cellb/LConn2
  Solar Cellc/LConn2 -- Solar Cellb/RConn1
  Solar Celld/LConn2 -- Solar Cellc/RConn1
  Solar Celle/LConn2 -- Solar Celld/RConn1
  Solar Cellf/LConn2 -- Solar Celle/RConn1
  +/RConn1 -- Solar Cella/LConn2
  -/RConn1 -- Solar Cellf/RConn1

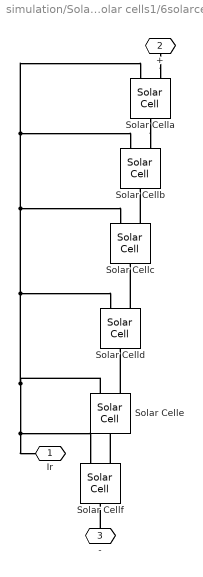
== system simulation/Solar module (72 cells)1/36 solarceel1/18 solar cells1/6solarcells ==
  Solar Cella : elec_lib/Sources/Solar Cell  prm=1  Isc=4.75 A  Voc=0.6 V  Is=1e-6 A  Is2=0 A  Iph=7.34 A  Ir0=1000 W/m^2  ec=1.6  N2=2  Rs=5.1e-3 Ohm  Rp=Inf Ohm  TIPH1=0.65e-3 1/K  EG=1.12 eV  TXIS1=3  TXIS2=3  TRS1=0  TRP1=0  Tmeas=25 C  TFIXED=25 C  LocalVarLogging=[]  thermal_mass=100 J/K  initial_temperature=25 C
  Solar Cellb : elec_lib/Sources/Solar Cell  prm=1  Isc=4.75 A  Voc=0.6 V  Is=1e-6 A  Is2=0 A  Iph=7.34 A  Ir0=1000 W/m^2  ec=1.6  N2=2  Rs=5.1e-3 Ohm  Rp=Inf Ohm  TIPH1=0.65e-3 1/K  EG=1.12 eV  TXIS1=3  TXIS2=3  TRS1=0  TRP1=0  Tmeas=25 C  TFIXED=25 C  LocalVarLogging=[]  thermal_mass=100 J/K  initial_temperature=25 C
  Solar Cellc : elec_lib/Sources/Solar Cell  prm=1  Isc=4.75 A  Voc=0.6 V  Is=1e-6 A  Is2=0 A  Iph=7.34 A  Ir0=1000 W/m^2  ec=1.6  N2=2  Rs=5.1e-3 Ohm  Rp=Inf Ohm  TIPH1=0.65e-3 1/K  EG=1.12 eV  TXIS1=3  TXIS2=3  TRS1=0  TRP1=0  Tmeas=25 C  TFIXED=25 C  LocalVarLogging=[]  thermal_mass=100 J/K  initial_temperature=25 C
  Solar Celld : elec_lib/Sources/Solar Cell  prm=1  Isc=4.75 A  Voc=0.6 V  Is=1e-6 A  Is2=0 A  Iph=7.34 A  Ir0=1000 W/m^2  ec=1.6  N2=2  Rs=5.1e-3 Ohm  Rp=Inf Ohm  TIPH1=0.65e-3 1/K  EG=1.12 eV  TXIS1=3  TXIS2=3  TRS1=0  TRP1=0  Tmeas=25 C  TFIXED=25 C  LocalVarLogging=[]  thermal_mass=100 J/K  initial_temperature=25 C
  Solar Celle : elec_lib/Sources/Solar Cell  prm=1  Isc=4.75 A  Voc=0.6 V  Is=1e-6 A  Is2=0 A  Iph=7.34 A  Ir0=1000 W/m^2  ec=1.6  N2=2  Rs=5.1e-3 Ohm  Rp=Inf Ohm  TIPH1=0.65e-3 1/K  EG=1.12 eV  TXIS1=3  TXIS2=3  TRS1=0  TRP1=0  Tmeas=25 C  TFIXED=25 C  LocalVarLogging=[]  thermal_mass=100 J/K  initial_temperature=25 C
  Solar Cellf : elec_lib/Sources/Solar Cell  prm=1  Isc=4.75 A  Voc=0.6 V  Is=1e-6 A  Is2=0 A  Iph=7.34 A  Ir0=1000 W/m^2  ec=1.6  N2=2  Rs=5.1e-3 Ohm  Rp=Inf Ohm  TIPH1=0.65e-3 1/K  EG=1.12 eV  TXIS1=3  TXIS2=3  TRS1=0  TRP1=0  Tmeas=25 C  TFIXED=25 C  LocalVarLogging=[]  thermal_mass=100 J/K  initial_temperature=25 C
  Ir : PMIOPort  Port=1  Side=Left
  + : PMIOPort  Port=2  Side=Right
  - : PMIOPort  Port=3  Side=Left
  connections:
  Solar Celle/LConn1 -- Solar Cellf/LConn1 -- Ir/RConn1 -- Solar Celld/LConn1 -- Solar Cellc/LConn1 -- Solar Cella/LConn1 -- Solar Cellb/LConn1
  Solar Cella/RConn1 -- Solar Cellb/LConn2
  Solar Cellc/LConn2 -- Solar Cellb/RConn1
  Solar Celld/LConn2 -- Solar Cellc/RConn1
  Solar Celle/LConn2 -- Solar Celld/RConn1
  Solar Cellf/LConn2 -- Solar Celle/RConn1
  +/RConn1 -- Solar Cella/LConn2
  -/RConn1 -- Solar Cellf/RConn1

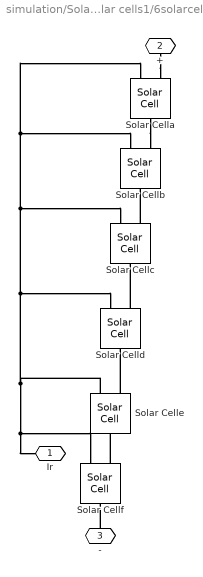
== system simulation/Solar module (72 cells)1/36 solarceel1/18 solar cells1/6solarcells1 ==
  Solar Cella : elec_lib/Sources/Solar Cell  prm=1  Isc=4.75 A  Voc=0.6 V  Is=1e-6 A  Is2=0 A  Iph=7.34 A  Ir0=1000 W/m^2  ec=1.6  N2=2  Rs=5.1e-3 Ohm  Rp=Inf Ohm  TIPH1=0.65e-3 1/K  EG=1.12 eV  TXIS1=3  TXIS2=3  TRS1=0  TRP1=0  Tmeas=25 C  TFIXED=25 C  LocalVarLogging=[]  thermal_mass=100 J/K  initial_temperature=25 C
  Solar Cellb : elec_lib/Sources/Solar Cell  prm=1  Isc=4.75 A  Voc=0.6 V  Is=1e-6 A  Is2=0 A  Iph=7.34 A  Ir0=1000 W/m^2  ec=1.6  N2=2  Rs=5.1e-3 Ohm  Rp=Inf Ohm  TIPH1=0.65e-3 1/K  EG=1.12 eV  TXIS1=3  TXIS2=3  TRS1=0  TRP1=0  Tmeas=25 C  TFIXED=25 C  LocalVarLogging=[]  thermal_mass=100 J/K  initial_temperature=25 C
  Solar Cellc : elec_lib/Sources/Solar Cell  prm=1  Isc=4.75 A  Voc=0.6 V  Is=1e-6 A  Is2=0 A  Iph=7.34 A  Ir0=1000 W/m^2  ec=1.6  N2=2  Rs=5.1e-3 Ohm  Rp=Inf Ohm  TIPH1=0.65e-3 1/K  EG=1.12 eV  TXIS1=3  TXIS2=3  TRS1=0  TRP1=0  Tmeas=25 C  TFIXED=25 C  LocalVarLogging=[]  thermal_mass=100 J/K  initial_temperature=25 C
  Solar Celld : elec_lib/Sources/Solar Cell  prm=1  Isc=4.75 A  Voc=0.6 V  Is=1e-6 A  Is2=0 A  Iph=7.34 A  Ir0=1000 W/m^2  ec=1.6  N2=2  Rs=5.1e-3 Ohm  Rp=Inf Ohm  TIPH1=0.65e-3 1/K  EG=1.12 eV  TXIS1=3  TXIS2=3  TRS1=0  TRP1=0  Tmeas=25 C  TFIXED=25 C  LocalVarLogging=[]  thermal_mass=100 J/K  initial_temperature=25 C
  Solar Celle : elec_lib/Sources/Solar Cell  prm=1  Isc=4.75 A  Voc=0.6 V  Is=1e-6 A  Is2=0 A  Iph=7.34 A  Ir0=1000 W/m^2  ec=1.6  N2=2  Rs=5.1e-3 Ohm  Rp=Inf Ohm  TIPH1=0.65e-3 1/K  EG=1.12 eV  TXIS1=3  TXIS2=3  TRS1=0  TRP1=0  Tmeas=25 C  TFIXED=25 C  LocalVarLogging=[]  thermal_mass=100 J/K  initial_temperature=25 C
  Solar Cellf : elec_lib/Sources/Solar Cell  prm=1  Isc=4.75 A  Voc=0.6 V  Is=1e-6 A  Is2=0 A  Iph=7.34 A  Ir0=1000 W/m^2  ec=1.6  N2=2  Rs=5.1e-3 Ohm  Rp=Inf Ohm  TIPH1=0.65e-3 1/K  EG=1.12 eV  TXIS1=3  TXIS2=3  TRS1=0  TRP1=0  Tmeas=25 C  TFIXED=25 C  LocalVarLogging=[]  thermal_mass=100 J/K  initial_temperature=25 C
  Ir : PMIOPort  Port=1  Side=Left
  + : PMIOPort  Port=2  Side=Right
  - : PMIOPort  Port=3  Side=Left
  connections:
  Solar Celle/LConn1 -- Solar Cellf/LConn1 -- Ir/RConn1 -- Solar Celld/LConn1 -- Solar Cellc/LConn1 -- Solar Cella/LConn1 -- Solar Cellb/LConn1
  Solar Cella/RConn1 -- Solar Cellb/LConn2
  Solar Cellc/LConn2 -- Solar Cellb/RConn1
  Solar Celld/LConn2 -- Solar Cellc/RConn1
  Solar Celle/LConn2 -- Solar Celld/RConn1
  Solar Cellf/LConn2 -- Solar Celle/RConn1
  +/RConn1 -- Solar Cella/LConn2
  -/RConn1 -- Solar Cellf/RConn1

== system simulation/Solar module (72 cells)1/36 solarceel1/18 solar cells1/6solarcells2 ==
  Solar Cella : elec_lib/Sources/Solar Cell  prm=1  Isc=4.75 A  Voc=0.6 V  Is=1e-6 A  Is2=0 A  Iph=7.34 A  Ir0=1000 W/m^2  ec=1.6  N2=2  Rs=5.1e-3 Ohm  Rp=Inf Ohm  TIPH1=0.65e-3 1/K  EG=1.12 eV  TXIS1=3  TXIS2=3  TRS1=0  TRP1=0  Tmeas=25 C  TFIXED=25 C  LocalVarLogging=[]  thermal_mass=100 J/K  initial_temperature=25 C
  Solar Cellb : elec_lib/Sources/Solar Cell  prm=1  Isc=4.75 A  Voc=0.6 V  Is=1e-6 A  Is2=0 A  Iph=7.34 A  Ir0=1000 W/m^2  ec=1.6  N2=2  Rs=5.1e-3 Ohm  Rp=Inf Ohm  TIPH1=0.65e-3 1/K  EG=1.12 eV  TXIS1=3  TXIS2=3  TRS1=0  TRP1=0  Tmeas=25 C  TFIXED=25 C  LocalVarLogging=[]  thermal_mass=100 J/K  initial_temperature=25 C
  Solar Cellc : elec_lib/Sources/Solar Cell  prm=1  Isc=4.75 A  Voc=0.6 V  Is=1e-6 A  Is2=0 A  Iph=7.34 A  Ir0=1000 W/m^2  ec=1.6  N2=2  Rs=5.1e-3 Ohm  Rp=Inf Ohm  TIPH1=0.65e-3 1/K  EG=1.12 eV  TXIS1=3  TXIS2=3  TRS1=0  TRP1=0  Tmeas=25 C  TFIXED=25 C  LocalVarLogging=[]  thermal_mass=100 J/K  initial_temperature=25 C
  Solar Celld : elec_lib/Sources/Solar Cell  prm=1  Isc=4.75 A  Voc=0.6 V  Is=1e-6 A  Is2=0 A  Iph=7.34 A  Ir0=1000 W/m^2  ec=1.6  N2=2  Rs=5.1e-3 Ohm  Rp=Inf Ohm  TIPH1=0.65e-3 1/K  EG=1.12 eV  TXIS1=3  TXIS2=3  TRS1=0  TRP1=0  Tmeas=25 C  TFIXED=25 C  LocalVarLogging=[]  thermal_mass=100 J/K  initial_temperature=25 C
  Solar Celle : elec_lib/Sources/Solar Cell  prm=1  Isc=4.75 A  Voc=0.6 V  Is=1e-6 A  Is2=0 A  Iph=7.34 A  Ir0=1000 W/m^2  ec=1.6  N2=2  Rs=5.1e-3 Ohm  Rp=Inf Ohm  TIPH1=0.65e-3 1/K  EG=1.12 eV  TXIS1=3  TXIS2=3  TRS1=0  TRP1=0  Tmeas=25 C  TFIXED=25 C  LocalVarLogging=[]  thermal_mass=100 J/K  initial_temperature=25 C
  Solar Cellf : elec_lib/Sources/Solar Cell  prm=1  Isc=4.75 A  Voc=0.6 V  Is=1e-6 A  Is2=0 A  Iph=7.34 A  Ir0=1000 W/m^2  ec=1.6  N2=2  Rs=5.1e-3 Ohm  Rp=Inf Ohm  TIPH1=0.65e-3 1/K  EG=1.12 eV  TXIS1=3  TXIS2=3  TRS1=0  TRP1=0  Tmeas=25 C  TFIXED=25 C  LocalVarLogging=[]  thermal_mass=100 J/K  initial_temperature=25 C
  Ir : PMIOPort  Port=1  Side=Left
  + : PMIOPort  Port=2  Side=Right
  - : PMIOPort  Port=3  Side=Left
  connections:
  Solar Celle/LConn1 -- Solar Cellf/LConn1 -- Ir/RConn1 -- Solar Celld/LConn1 -- Solar Cellc/LConn1 -- Solar Cella/LConn1 -- Solar Cellb/LConn1
  Solar Cella/RConn1 -- Solar Cellb/LConn2
  Solar Cellc/LConn2 -- Solar Cellb/RConn1
  Solar Celld/LConn2 -- Solar Cellc/RConn1
  Solar Celle/LConn2 -- Solar Celld/RConn1
  Solar Cellf/LConn2 -- Solar Celle/RConn1
  +/RConn1 -- Solar Cella/LConn2
  -/RConn1 -- Solar Cellf/RConn1
